simulink model "cyclicNetwork_3"  (Simulink 7.5)
settings: Solver=ode45  StartTime=0.0  StopTime=30.0  RelTol=1e-3
settings Model: Creator=james  LastModifiedBy=james

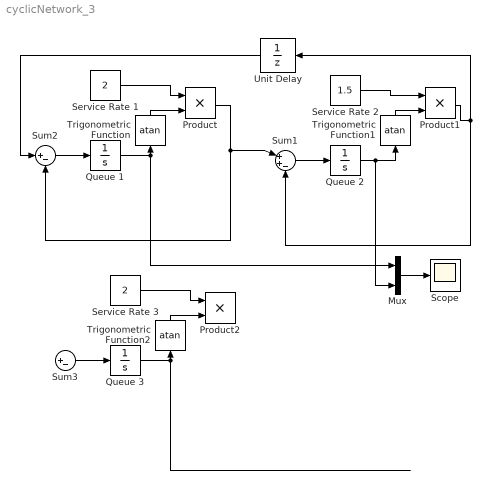
== system cyclicNetwork_3 ==
  Mux : Mux  Inputs=2
  Product : Product  OutDataType=fixdt(1, 16)  OutScaling=2^0  RndMeth=Zero
  Product1 : Product  OutDataType=fixdt(1, 16)  OutScaling=2^0  RndMeth=Zero
  Product2 : Product  OutDataType=fixdt(1, 16)  OutScaling=2^0  RndMeth=Zero
  Queue 1 : Integrator  InitialCondition=10  LimitOutput=on  LowerSaturationLimit=0
  Queue 2 : Integrator  LimitOutput=on  LowerSaturationLimit=0
  Queue 3 : Integrator  InitialCondition=10  LimitOutput=on  LowerSaturationLimit=0
  Scope : Scope
  Service Rate 1 : Constant  Value=2  OutDataType=fixdt(1, 16)  OutScaling=2^0
  Service Rate 2 : Constant  Value=1.5  OutDataType=fixdt(1, 16)  OutScaling=2^0
  Service Rate 3 : Constant  Value=2  OutDataType=fixdt(1, 16)  OutScaling=2^0
  Sum1 : Sum  Inputs=|++-  OutDataType=fixdt(1, 16)  OutScaling=2^0
  Sum2 : Sum  Inputs=|+-  OutDataType=fixdt(1, 16)  OutScaling=2^0
  Sum3 : Sum  Inputs=|+-  OutDataType=fixdt(1, 16)  OutScaling=2^0
  Trigonometric Function : Trigonometry  Operator=atan
  Trigonometric Function1 : Trigonometry  Operator=atan
  Trigonometric Function2 : Trigonometry  Operator=atan
  Unit Delay : UnitDelay  SampleTime=-1
  wires:
  Queue 2/1 -> Mux/2, Trigonometric Function1/1
  Sum1/1 -> Queue 2/1
  Product1/1 -> Unit Delay/1, Sum1/3
  Service Rate 1/1 -> Product/1
  Queue 1/1 -> Mux/1, Trigonometric Function/1
  Sum2/1 -> Queue 1/1
  Product/1 -> Sum2/2, Sum1/1
  Mux/1 -> Scope/1
  Unit Delay/1 -> Sum2/1
  Trigonometric Function/1 -> Product/2
  Service Rate 2/1 -> Product1/1
  Trigonometric Function1/1 -> Product1/2
  Service Rate 3/1 -> Product2/1
  Queue 3/1 -> Trigonometric Function2/1
  Sum3/1 -> Queue 3/1
  ? -> Sum3/2
  Trigonometric Function2/1 -> Product2/2
